simulink model "soc_dvbs2_fpga"  (R2025b)
settings: Solver=FixedStepDiscrete  StartTime=0.0  StopTime=0  RelTol=1e-3
InitFcn:
  | soc_dvbs2_init;
values from neighbouring files (symbols this model uses):
  Rsym = 4e6    (= 4000000)    [soc_dvbs2_init.m]
  soc_dvbs2_txPacketBits = [1 1 0 1 0 1 1 1 0 1 1 1 ... (2972 elements, 2972x1)]    [soc_dvbs2_txPacketBits.mat]
  syncWord = (dec2bin(hex2dec('AC')) - '0').'    [soc_dvbs2_init.m]
  txDataOut = txobj(frameBits(:))    [soc_dvbs2_init.m]
  txFiltCoeff = txobj.pTxFilterCoeff    [soc_dvbs2_init.m]
undefined symbols (not defined in the file or in its folder): Add, coefficientsLog, coefficientsSqrt1, coefficientsSqrt2, dataBits, designMultirateFIR, noisePow, NumBits1, NumBits2, seedsURNG1, seedsURNG2, Shift, Slope1, Slope2, soc_dvbs2_designFIRFilter, txDataOutS1, txDataOutS10, txDataOutS12, txDataOutS13, txDataOutS14, txDataOutS15, txDataOutS16, txDataOutS18, txDataOutS19, txDataOutS2, txDataOutS20, txDataOutS21, txDataOutS22, txDataOutS24, txDataOutS25, txDataOutS26, txDataOutS27, txDataOutS3, txDataOutS4, txDataOutS5, txDataOutS6, txDataOutS7, txDataOutS8, txDataOutS9
libraries: simulink x214, hdlsllib x211, dspsigops x22, dsphdlfiltering2 x8, dsphdlsigops2 x5, commseqgen3 x5, dsphdlmathfun2 x3, hwlogicconnlib x2, whdledac x2, commhdlcrc x2, whdlutilities x1, whdlmod x1
(part 9 of 12)

== system soc_dvbs2_fpga/DVBS2/DVBS2 TxRx/DVB-S2 HDL Receiver/Synchronizer and PL Header Decoder/Time Frequency and Coarse Phase Synchronizer/Coarse Phase Synchronizer/Coarse Phase Corrector/Reciprocal/Function Impl ==
  switch : Inport
  LUTAddr : Inport  Port=2
  Delay{6..8,10,15..16} (6 alike) : Delay
  Delay9 : Delay  DelayLength=1
  LUT1 : LookupNDDirect  NumberOfTableDimensions=1  Table=LUT(:,1)  DiagnosticForOutOfRangeInput=Error
  LUT2 : LookupNDDirect  NumberOfTableDimensions=1  Table=LUT(:,2)  DiagnosticForOutOfRangeInput=Error
  Multiport Switch : MultiPortSwitch  DataPortOrder=Zero-based contiguous  Inputs=2  zeroidx=on  SaturateOnIntegerOverflow=off  InputSameDT=off
  functionValues : Outport
  wires:
  LUTAddr/1 -> Delay7/1, Delay6/1
  Delay15/1 -> Multiport Switch/2
  Delay16/1 -> Multiport Switch/3
  Delay10/1 -> Multiport Switch/1
  Delay9/1 -> functionValues/1
  LUT2/1 -> Delay15/1
  LUT1/1 -> Delay16/1
  switch/1 -> Delay8/1
  Delay8/1 -> Delay10/1
  Delay7/1 -> LUT2/1
  Delay6/1 -> LUT1/1
  Multiport Switch/1 -> Delay9/1

== system soc_dvbs2_fpga/DVBS2/DVBS2 TxRx/DVB-S2 HDL Receiver/Synchronizer and PL Header Decoder/Time Frequency and Coarse Phase Synchronizer/Fine Frequency Synchronizer/Modified L and R Algorithm/L and R Algorithm 18 point/Compute R(m) for 1 to 6 ==
  z : Inport
  zvalid : Inport  Port=2
  Add2 : Sum  Inputs=++++++
  Compute R(m)_1 : Subsystem  mask{m=m(1), N=config.nPilot}
      mask prompts: m "m value :"; N "N value :"
      mask init:
      | validateattributes(N,{'numeric'},{'finite','positive','integer'})
      | validateattributes(m,{'numeric'},{'finite','positive','integer','>=',1,'<=',N-1})
      | MulDivFactor = fi(1/(N-m),0,16);
  Compute R(m)_2 : Subsystem  mask{m=m(2), N=config.nPilot}
      mask prompts: m "m value :"; N "N value :"
      mask init:
      | validateattributes(N,{'numeric'},{'finite','positive','integer'})
      | validateattributes(m,{'numeric'},{'finite','positive','integer','>=',1,'<=',N-1})
      | MulDivFactor = fi(1/(N-m),0,16);
  Compute R(m)_3 : Subsystem  mask{m=m(3), N=config.nPilot}
      mask prompts: m "m value :"; N "N value :"
      mask init:
      | validateattributes(N,{'numeric'},{'finite','positive','integer'})
      | validateattributes(m,{'numeric'},{'finite','positive','integer','>=',1,'<=',N-1})
      | MulDivFactor = fi(1/(N-m),0,16);
  Compute R(m)_4 : Subsystem  mask{m=m(4), N=config.nPilot}
      mask prompts: m "m value :"; N "N value :"
      mask init:
      | validateattributes(N,{'numeric'},{'finite','positive','integer'})
      | validateattributes(m,{'numeric'},{'finite','positive','integer','>=',1,'<=',N-1})
      | MulDivFactor = fi(1/(N-m),0,16);
  Compute R(m)_5 : Subsystem  mask{m=m(5), N=config.nPilot}
      mask prompts: m "m value :"; N "N value :"
      mask init:
      | validateattributes(N,{'numeric'},{'finite','positive','integer'})
      | validateattributes(m,{'numeric'},{'finite','positive','integer','>=',1,'<=',N-1})
      | MulDivFactor = fi(1/(N-m),0,16);
  Compute R(m)_6 : Subsystem  mask{m=m(6), N=config.nPilot}
      mask prompts: m "m value :"; N "N value :"
      mask init:
      | validateattributes(N,{'numeric'},{'finite','positive','integer'})
      | validateattributes(m,{'numeric'},{'finite','positive','integer','>=',1,'<=',N-1})
      | MulDivFactor = fi(1/(N-m),0,16);
  Delay{1..7} (7 alike) : Delay
  sum : Outport
  wires:
  z/1 -> Compute R(m)_1/1(z), Compute R(m)_5/1(z), Compute R(m)_6/1(z), Compute R(m)_4/1(z), Compute R(m)_3/1(z), Compute R(m)_2/1(z)
  Delay3/1 -> Add2/1
  Delay7/1 -> sum/1
  Delay6/1 -> Add2/6
  Delay5/1 -> Add2/5
  Delay4/1 -> Add2/4
  Delay2/1 -> Add2/3
  Delay1/1 -> Add2/2
  zvalid/1 -> Compute R(m)_1/2(zvalid), Compute R(m)_5/2(zvalid), Compute R(m)_6/2(zvalid), Compute R(m)_4/2(zvalid), Compute R(m)_3/2(zvalid), Compute R(m)_2/2(zvalid)
  Compute R(m)_6/1(Out1) -> Delay6/1
  Compute R(m)_5/1(Out1) -> Delay5/1
  Compute R(m)_4/1(Out1) -> Delay4/1
  Compute R(m)_3/1(Out1) -> Delay2/1
  Compute R(m)_2/1(Out1) -> Delay1/1
  Compute R(m)_1/1(Out1) -> Delay3/1
  Add2/1 -> Delay7/1

== system soc_dvbs2_fpga/DVBS2/DVBS2 TxRx/DVB-S2 HDL Receiver/Synchronizer and PL Header Decoder/Time Frequency and Coarse Phase Synchronizer/Fine Frequency Synchronizer/Modified L and R Algorithm/L and R Algorithm 18 point/Compute R(m) for 13 to 18 ==
  z : Inport
  zvalid : Inport  Port=2
  Add2 : Sum  Inputs=++++++
  Compute R(m)_1 : Subsystem  mask{m=m(1), N=config.nPilot}
      mask prompts: m "m value :"; N "N value :"
      mask init:
      | validateattributes(N,{'numeric'},{'finite','positive','integer'})
      | validateattributes(m,{'numeric'},{'finite','positive','integer','>=',1,'<=',N-1})
      | MulDivFactor = fi(1/(N-m),0,16);
  Compute R(m)_2 : Subsystem  mask{m=m(2), N=config.nPilot}
      mask prompts: m "m value :"; N "N value :"
      mask init:
      | validateattributes(N,{'numeric'},{'finite','positive','integer'})
      | validateattributes(m,{'numeric'},{'finite','positive','integer','>=',1,'<=',N-1})
      | MulDivFactor = fi(1/(N-m),0,16);
  Compute R(m)_3 : Subsystem  mask{m=m(3), N=config.nPilot}
      mask prompts: m "m value :"; N "N value :"
      mask init:
      | validateattributes(N,{'numeric'},{'finite','positive','integer'})
      | validateattributes(m,{'numeric'},{'finite','positive','integer','>=',1,'<=',N-1})
      | MulDivFactor = fi(1/(N-m),0,16);
  Compute R(m)_4 : Subsystem  mask{m=m(4), N=config.nPilot}
      mask prompts: m "m value :"; N "N value :"
      mask init:
      | validateattributes(N,{'numeric'},{'finite','positive','integer'})
      | validateattributes(m,{'numeric'},{'finite','positive','integer','>=',1,'<=',N-1})
      | MulDivFactor = fi(1/(N-m),0,16);
  Compute R(m)_5 : Subsystem  mask{m=m(5), N=config.nPilot}
      mask prompts: m "m value :"; N "N value :"
      mask init:
      | validateattributes(N,{'numeric'},{'finite','positive','integer'})
      | validateattributes(m,{'numeric'},{'finite','positive','integer','>=',1,'<=',N-1})
      | MulDivFactor = fi(1/(N-m),0,16);
  Compute R(m)_6 : Subsystem  mask{m=m(6), N=config.nPilot}
      mask prompts: m "m value :"; N "N value :"
      mask init:
      | validateattributes(N,{'numeric'},{'finite','positive','integer'})
      | validateattributes(m,{'numeric'},{'finite','positive','integer','>=',1,'<=',N-1})
      | MulDivFactor = fi(1/(N-m),0,16);
  Delay{1..7} (7 alike) : Delay
  sum : Outport
  wires:
  z/1 -> Compute R(m)_1/1(z), Compute R(m)_5/1(z), Compute R(m)_6/1(z), Compute R(m)_4/1(z), Compute R(m)_3/1(z), Compute R(m)_2/1(z)
  Delay3/1 -> Add2/1
  Delay7/1 -> sum/1
  Delay6/1 -> Add2/6
  Delay5/1 -> Add2/5
  Delay4/1 -> Add2/4
  Delay2/1 -> Add2/3
  Delay1/1 -> Add2/2
  zvalid/1 -> Compute R(m)_1/2(zvalid), Compute R(m)_5/2(zvalid), Compute R(m)_6/2(zvalid), Compute R(m)_4/2(zvalid), Compute R(m)_3/2(zvalid), Compute R(m)_2/2(zvalid)
  Compute R(m)_6/1(Out1) -> Delay6/1
  Compute R(m)_5/1(Out1) -> Delay5/1
  Compute R(m)_4/1(Out1) -> Delay4/1
  Compute R(m)_3/1(Out1) -> Delay2/1
  Compute R(m)_2/1(Out1) -> Delay1/1
  Compute R(m)_1/1(Out1) -> Delay3/1
  Add2/1 -> Delay7/1

== system soc_dvbs2_fpga/DVBS2/DVBS2 TxRx/DVB-S2 HDL Receiver/Synchronizer and PL Header Decoder/Time Frequency and Coarse Phase Synchronizer/Fine Frequency Synchronizer/Modified L and R Algorithm/L and R Algorithm 18 point/Compute R(m) for 7 to 12 ==
  z : Inport
  zvalid : Inport  Port=2
  Add2 : Sum  Inputs=++++++
  Compute R(m)_1 : Subsystem  mask{m=m(1), N=config.nPilot}
      mask prompts: m "m value :"; N "N value :"
      mask init:
      | validateattributes(N,{'numeric'},{'finite','positive','integer'})
      | validateattributes(m,{'numeric'},{'finite','positive','integer','>=',1,'<=',N-1})
      | MulDivFactor = fi(1/(N-m),0,16);
  Compute R(m)_2 : Subsystem  mask{m=m(2), N=config.nPilot}
      mask prompts: m "m value :"; N "N value :"
      mask init:
      | validateattributes(N,{'numeric'},{'finite','positive','integer'})
      | validateattributes(m,{'numeric'},{'finite','positive','integer','>=',1,'<=',N-1})
      | MulDivFactor = fi(1/(N-m),0,16);
  Compute R(m)_3 : Subsystem  mask{m=m(3), N=config.nPilot}
      mask prompts: m "m value :"; N "N value :"
      mask init:
      | validateattributes(N,{'numeric'},{'finite','positive','integer'})
      | validateattributes(m,{'numeric'},{'finite','positive','integer','>=',1,'<=',N-1})
      | MulDivFactor = fi(1/(N-m),0,16);
  Compute R(m)_4 : Subsystem  mask{m=m(4), N=config.nPilot}
      mask prompts: m "m value :"; N "N value :"
      mask init:
      | validateattributes(N,{'numeric'},{'finite','positive','integer'})
      | validateattributes(m,{'numeric'},{'finite','positive','integer','>=',1,'<=',N-1})
      | MulDivFactor = fi(1/(N-m),0,16);
  Compute R(m)_5 : Subsystem  mask{m=m(5), N=config.nPilot}
      mask prompts: m "m value :"; N "N value :"
      mask init:
      | validateattributes(N,{'numeric'},{'finite','positive','integer'})
      | validateattributes(m,{'numeric'},{'finite','positive','integer','>=',1,'<=',N-1})
      | MulDivFactor = fi(1/(N-m),0,16);
  Compute R(m)_6 : Subsystem  mask{m=m(6), N=config.nPilot}
      mask prompts: m "m value :"; N "N value :"
      mask init:
      | validateattributes(N,{'numeric'},{'finite','positive','integer'})
      | validateattributes(m,{'numeric'},{'finite','positive','integer','>=',1,'<=',N-1})
      | MulDivFactor = fi(1/(N-m),0,16);
  Delay{1..7} (7 alike) : Delay
  sum : Outport
  wires:
  Add2/1 -> Delay7/1
  Compute R(m)_1/1(Out1) -> Delay3/1
  Compute R(m)_2/1(Out1) -> Delay1/1
  Compute R(m)_3/1(Out1) -> Delay2/1
  Compute R(m)_4/1(Out1) -> Delay4/1
  Compute R(m)_5/1(Out1) -> Delay5/1
  Compute R(m)_6/1(Out1) -> Delay6/1
  zvalid/1 -> Compute R(m)_2/2(zvalid), Compute R(m)_3/2(zvalid), Compute R(m)_4/2(zvalid), Compute R(m)_6/2(zvalid), Compute R(m)_5/2(zvalid), Compute R(m)_1/2(zvalid)
  Delay1/1 -> Add2/2
  Delay2/1 -> Add2/3
  Delay4/1 -> Add2/4
  Delay5/1 -> Add2/5
  Delay6/1 -> Add2/6
  Delay7/1 -> sum/1
  Delay3/1 -> Add2/1
  z/1 -> Compute R(m)_2/1(z), Compute R(m)_3/1(z), Compute R(m)_4/1(z), Compute R(m)_6/1(z), Compute R(m)_5/1(z), Compute R(m)_1/1(z)

== system soc_dvbs2_fpga/DVBS2/DVBS2 TxRx/DVB-S2 HDL Receiver/Synchronizer and PL Header Decoder/Time Frequency and Coarse Phase Synchronizer/Time and Coarse Frequency Synchronizer/Coarse Frequency Estimator/Frequency Error Detector/Complex Multiplier ==
  In1 : Inport
  In2 : Inport  Port=2
  AddADn : Sum  Inputs=++|  OutDataTypeStr=Inherit: Same as first input
  AddAUp : Sum  Inputs=|+-  OutDataTypeStr=Inherit: Same as first input
  AddBCtr : Sum  Inputs=+|+
  AddBDn : Sum  Inputs=|+-
  AddBUp : Sum  Inputs=++|
  Complex to Real-Imag : ComplexToRealImag
  Complex to Real-Imag1 : ComplexToRealImag
  Delay{1..5,8..20} (18 alike) : Delay  DelayLength=1
  Delay{6..7,21..27} (9 alike) : Delay
  Product : Product
  Product1 : Product
  Product2 : Product
  Real-Imag to Complex : RealImagToComplex
  Out1 : Outport  VectorParamsAs1DForOutWhenUnconnected=off
  wires:
  Delay27/1 -> Delay18/1
  Delay26/1 -> Delay17/1
  Delay25/1 -> Delay16/1
  Delay24/1 -> Product2/2
  Delay23/1 -> Product2/1
  Delay22/1 -> Product1/2
  Delay21/1 -> Product1/1
  Delay7/1 -> Product/2
  Delay6/1 -> Product/1
  Delay13/1 -> AddBCtr/2, Delay4/1
  Delay12/1 -> Delay3/1
  Delay11/1 -> AddBCtr/1, Delay1/1
  In2/1 -> Complex to Real-Imag1/1
  In1/1 -> Complex to Real-Imag/1
  Product2/1 -> Delay27/1
  Product1/1 -> Delay26/1
  Product/1 -> Delay25/1
  Complex to Real-Imag1/1 -> [RE2]
  Complex to Real-Imag1/2 -> [IM2]
  [IM2] -> Delay10/1
  [RE2] -> Delay9/1
  Complex to Real-Imag/1 -> Delay11/1
  AddBUp/1 -> Delay8/1
  [RE2] -> Delay14/1
  [IM2] -> Delay15/1
  AddBDn/1 -> Delay5/1
  Complex to Real-Imag/2 -> Delay13/1
  AddBCtr/1 -> Delay2/1
  [IM2] -> Delay12/1
  AddADn/1 -> Delay20/1
  AddAUp/1 -> Delay19/1
  Real-Imag to Complex/1 -> Out1/1
  Delay5/1 -> Delay24/1
  Delay4/1 -> Delay23/1
  Delay3/1 -> Delay22/1
  Delay2/1 -> Delay21/1
  Delay8/1 -> Delay6/1
  Delay9/1 -> AddBUp/1
  Delay10/1 -> AddBUp/2
  Delay14/1 -> AddBDn/1
  Delay15/1 -> AddBDn/2
  Delay16/1 -> AddAUp/1
  Delay17/1 -> AddADn/1, AddAUp/2
  Delay18/1 -> AddADn/2
  Delay19/1 -> Real-Imag to Complex/1
  Delay20/1 -> Real-Imag to Complex/2
  Delay1/1 -> Delay7/1

== system soc_dvbs2_fpga/DVBS2/DVBS2 TxRx/DVB-S2 HDL Receiver/Synchronizer and PL Header Decoder/Time Frequency and Coarse Phase Synchronizer/Time and Coarse Frequency Synchronizer/Frame Synchronizer/Correlator/Moving Sum ==
  scaled1 : Inport
  scaled2 : Inport  Port=2
  validIn : Inport  Port=3
  Add : Sum  Inputs=|+-  OutDataTypeStr=Inherit: Same as first input
  Add1 : Sum  Inputs=|++  OutDataTypeStr=Inherit: Same as first input
  Add2 : Sum  Inputs=|+-  OutDataTypeStr=Inherit: Same as first input
  Add3 : Sum  Inputs=|++  OutDataTypeStr=Inherit: Same as first input
  Delay : Delay  DelayLength=length(config.refSOF)  ShowEnablePort=on
      settings: InputPortMap=u0,e6
  Delay1 : Delay  DelayLength=length(config.refPLSC)  ShowEnablePort=on
      settings: InputPortMap=u0,e6
  Delay11 : Delay  DelayLength=70
  Delay14 : Delay  DelayLength=1  ShowEnablePort=on
      settings: InputPortMap=u0,e6
  Delay2 : Delay  DelayLength=1  ShowEnablePort=on
      settings: InputPortMap=u0,e6
  Delay3 : Delay  DelayLength=length(config.refPLSC) - length(config.refSOF)  ShowEnablePort=on
      settings: InputPortMap=u0,e6
  Delay4 : Delay  DelayLength=70
  E1 : Outport
  E2 : Outport  Port=2
  wires:
  Delay4/1 -> E2/1
  Delay11/1 -> E1/1
  Delay3/1 -> Delay11/1
  Delay2/1 -> Add3/2
  scaled1/1 -> Add/1, Delay/1
  Delay1/1 -> Add2/2
  Add2/1 -> Add3/1
  Delay14/1 -> Add1/2
  Delay/1 -> Add/2
  Add3/1 -> Delay4/1, Delay2/1
  validIn/1 -> Delay14/2, Delay3/2, Delay/2, Delay1/2, Delay2/2
  Add1/1 -> Delay14/1, Delay3/1
  scaled2/1 -> Delay1/1, Add2/1
  Add/1 -> Add1/1

== system soc_dvbs2_fpga/DVBS2/DVBS2 TxRx/DVB-S2 HDL Receiver/Synchronizer and PL Header Decoder/Time Frequency and Coarse Phase Synchronizer/Time and Coarse Frequency Synchronizer/Frame Synchronizer/Correlator/PLSC Correlator ==
  dataIn : Inport
  validIn : Inport  Port=2
  Data Type Conversion : DataTypeConversion  OutDataTypeStr=fixdt(1,18,15)  SaturateOnIntegerOverflow=off  RndMeth=Floor
  Delay : Delay  DelayLength=partlySerialExtraDelay
  Delay1 : Delay  DelayLength=partlySerialExtraDelay
  Delay3 : Delay  DelayLength=adjustDelay
  Discrete FIR Filter : dsphdlfiltering2/Discrete FIR Filter  NumeratorSource=Property  Numerator=coefs  NumeratorPrototype=[]  FilterStructure=Partly serial systolic  SerializationOption=Minimum number of cycles between valid input samples  NumCycles=shareFactor  NumberOfMultipliers=2  SimulateUsing=Code generation  roundingMode=Floor  overflowMode=off  CoefficientsDataTypeStr=Inherit: Same word length as input  OutputDataTypeStr=Inherit: Same word length as input  ResetInputPort=off  HDLGlobalReset=off  CoeffMultiplier=Multiplier  UseMultForPow2Coeff=on  FrameInputSymmOptim=off
  Downsample : DownSample  N=shareFactor  RateOptions=Allow multirate processing
  Terminator : Terminator
  Unit Delay Enabled Synchronous : hdlsllib/Discrete/Unit Delay Enabled Synchronous  InitialCondition=0.0  SampleTime=-1
  Upsample : dspsigops/Upsample  FactorSource=Dialog parameter  N=shareFactor  Nmax=16  phase=0  RateOptions=Allow multirate processing  ic=0  mode=Unused parameter value
  Upsample1 : dspsigops/Upsample  FactorSource=Dialog parameter  N=shareFactor  Nmax=16  phase=0  RateOptions=Allow multirate processing  ic=0  mode=Unused parameter value
  dataOut : Outport
  wires:
  Downsample/1 -> Delay3/1
  Delay1/1 -> Unit Delay Enabled Synchronous/2
  Upsample1/1 -> Discrete FIR Filter/2
  Discrete FIR Filter/1 -> Delay/1
  Delay/1 -> Unit Delay Enabled Synchronous/1
  Discrete FIR Filter/2 -> Delay1/1
  Unit Delay Enabled Synchronous/1 -> Downsample/1
  Upsample/1 -> Discrete FIR Filter/1
  dataIn/1 -> Upsample/1
  validIn/1 -> Upsample1/1
  Delay3/1 -> Data Type Conversion/1
  Discrete FIR Filter/3 -> Terminator/1
  Data Type Conversion/1 -> dataOut/1

== system soc_dvbs2_fpga/DVBS2/DVBS2 TxRx/DVB-S2 HDL Receiver/Synchronizer and PL Header Decoder/Time Frequency and Coarse Phase Synchronizer/Time and Coarse Frequency Synchronizer/Frame Synchronizer/Correlator/SOF Correlator ==
  dataIn : Inport
  validIn : Inport  Port=2
  Data Type Conversion : DataTypeConversion  OutDataTypeStr=fixdt(1,18,15)  SaturateOnIntegerOverflow=off  RndMeth=Floor
  Delay : Delay  DelayLength=partlySerialExtraDelay
  Delay1 : Delay  DelayLength=partlySerialExtraDelay
  Delay3 : Delay  DelayLength=adjustDelay
  Discrete FIR Filter : dsphdlfiltering2/Discrete FIR Filter  NumeratorSource=Property  Numerator=coefs  NumeratorPrototype=[]  FilterStructure=Partly serial systolic  SerializationOption=Minimum number of cycles between valid input samples  NumCycles=shareFactor  NumberOfMultipliers=2  SimulateUsing=Code generation  roundingMode=Floor  overflowMode=off  CoefficientsDataTypeStr=Inherit: Same word length as input  OutputDataTypeStr=Inherit: Same word length as input  ResetInputPort=off  HDLGlobalReset=off  CoeffMultiplier=Multiplier  UseMultForPow2Coeff=on  FrameInputSymmOptim=off
  Downsample : DownSample  N=shareFactor  RateOptions=Allow multirate processing
  Terminator : Terminator
  Unit Delay Enabled Synchronous : hdlsllib/Discrete/Unit Delay Enabled Synchronous  InitialCondition=0.0  SampleTime=-1
  Upsample : dspsigops/Upsample  FactorSource=Dialog parameter  N=shareFactor  Nmax=16  phase=0  RateOptions=Allow multirate processing  ic=0  mode=Unused parameter value
  Upsample1 : dspsigops/Upsample  FactorSource=Dialog parameter  N=shareFactor  Nmax=16  phase=0  RateOptions=Allow multirate processing  ic=0  mode=Unused parameter value
  dataOut : Outport
  wires:
  Data Type Conversion/1 -> dataOut/1
  Discrete FIR Filter/3 -> Terminator/1
  Delay3/1 -> Data Type Conversion/1
  validIn/1 -> Upsample1/1
  dataIn/1 -> Upsample/1
  Upsample/1 -> Discrete FIR Filter/1
  Unit Delay Enabled Synchronous/1 -> Downsample/1
  Discrete FIR Filter/2 -> Delay1/1
  Delay/1 -> Unit Delay Enabled Synchronous/1
  Discrete FIR Filter/1 -> Delay/1
  Upsample1/1 -> Discrete FIR Filter/2
  Delay1/1 -> Unit Delay Enabled Synchronous/2
  Downsample/1 -> Delay3/1

== system soc_dvbs2_fpga/DVBS2/DVBS2 TxRx/DVB-S2 HDL Receiver/Synchronizer and PL Header Decoder/Time Frequency and Coarse Phase Synchronizer/Time and Coarse Frequency Synchronizer/Frame Synchronizer/Pilot and Sync Pulse Indicator/No HDL Correlation Value ==
  PeakValueWithPilots : Inport
  In1 : Inport  Port=2
  PeakValueWithoutPilots : Inport  Port=3
  Delay27 : Delay  DelayLength=1
  Delay28 : Delay  DelayLength=1
  Switch : Switch  Criteria=u2 ~= 0  SaturateOnIntegerOverflow=off  InputSameDT=off
  Terminator : Terminator
  wires:
  PeakValueWithoutPilots/1 -> Delay28/1
  Delay28/1 -> Switch/3
  In1/1 -> Switch/2
  Delay27/1 -> Switch/1
  Switch/1 -> Terminator/1
  PeakValueWithPilots/1 -> Delay27/1

== system soc_dvbs2_fpga/DVBS2/DVBS2 TxRx/DVB-S2 HDL Receiver/Synchronizer and PL Header Decoder/Time Frequency and Coarse Phase Synchronizer/Time and Coarse Frequency Synchronizer/PL Data Descrambler and Pilot Valid Indicator/PL Data Descrambler/PL Scrambler Gold Sequence Generator ==
  reset : Inport
  validIn : Inport  Port=2
  Bit Concat : hdlsllib/Logic and Bit Operations/Bit Concat  numInputs=2
  Delay{,3..4,10,12..15} (8 alike) : Delay  DelayLength=1
  Delay{1..2,5..9,11} (8 alike) : Delay
  Logical Operator : Logic  Operator=XOR  AllPortsSameDT=off  OutDataTypeStr=boolean
  Logical Operator1 : Logic  Operator=XOR  AllPortsSameDT=off  OutDataTypeStr=boolean
  Logical Operator2 : Logic  Operator=OR  AllPortsSameDT=off  OutDataTypeStr=boolean
  Subsystem : Subsystem
  dataOut : Outport
  validOut : Outport  Port=2
  wires:
  Delay15/1 -> validOut/1
  Delay14/1 -> dataOut/1
  Delay13/1 -> Delay15/1
  Delay12/1 -> Bit Concat/2
  Delay10/1 -> Bit Concat/1
  Delay9/1 -> Logical Operator/2
  Delay8/1 -> Logical Operator/1
  Delay7/1 -> Logical Operator1/2
  Delay6/1 -> Logical Operator1/1
  Delay5/1 -> Delay13/1
  Delay4/1 -> Delay2/1, Logical Operator2/1
  Delay3/1 -> Delay/1
  Delay2/1 -> Delay5/1
  Delay1/1 -> Subsystem/Enable
  Delay11/1 -> Subsystem/1(reset)
  Delay/1 -> Logical Operator2/2, Delay11/1
  validIn/1 -> Delay4/1
  Logical Operator1/1 -> Delay10/1
  Logical Operator/1 -> Delay12/1
  Bit Concat/1 -> Delay14/1
  reset/1 -> Delay3/1
  Subsystem/1(xMnp131072) -> Delay6/1
  Subsystem/2(yM131072) -> Delay7/1
  Subsystem/3(xMn) -> Delay8/1
  Subsystem/4(yM0) -> Delay9/1
  Logical Operator2/1 -> Delay1/1

== system soc_dvbs2_fpga/DVBS2/DVBS2 TxRx/DVB-S2 HDL Receiver/Synchronizer and PL Header Decoder/Time Frequency and Coarse Phase Synchronizer/Time and Coarse Frequency Synchronizer/Symbol Synchronizer/Gardner TED/GTED ==
  In1 : Inport
  Add : Sum
  Add1 : Sum  Inputs=+-
  Add2 : Sum  Inputs=+-
  Complex to Real-Imag : ComplexToRealImag
  Delay{,1..7} (8 alike) : Delay  DelayLength=1
  Delay{8..13} (6 alike) : Delay
  Product : Product
  Product1 : Product
  Out1 : Outport
  wires:
  Delay13/1 -> Add/2
  Delay12/1 -> Product1/2
  Delay11/1 -> Product1/1
  Delay10/1 -> Add/1
  Delay9/1 -> Product/2
  Delay8/1 -> Product/1
  Complex to Real-Imag/2 -> Delay4/1, Add2/2
  Delay7/1 -> Add2/1
  Delay4/1 -> Delay5/1
  Delay6/1 -> Delay7/1
  Add2/1 -> Delay12/1
  Delay5/1 -> Delay6/1, Delay11/1
  Delay1/1 -> Delay8/1, Delay2/1
  Add1/1 -> Delay9/1
  Delay2/1 -> Delay3/1
  Delay/1 -> Delay1/1
  Delay3/1 -> Add1/1
  Complex to Real-Imag/1 -> Delay/1, Add1/2
  In1/1 -> Complex to Real-Imag/1
  Add/1 -> Out1/1
  Product1/1 -> Delay13/1
  Product/1 -> Delay10/1

== system soc_dvbs2_fpga/DVBS2/DVBS2 TxRx/DVB-S2 HDL Receiver/Synchronizer and PL Header Decoder/Time Frequency and Coarse Phase Synchronizer/Time and Coarse Frequency Synchronizer/Symbol Synchronizer/Rate Handle/FIFO ==
  data : Inport
  push : Inport  Port=2
  pop : Inport  Port=3
  Delay1 : Delay  DelayLength=1
  Delay2 : Delay  DelayLength=1
  HDL Counter : hdlsllib/Sources/HDL Counter  CountType=Count limited  CountInit=0  CountStep=1  CountMax=1024-1  CountFromType=Initial value  CountFrom=0  CountResetPort=off  CountLoadPort=off  CountEnbPort=on  CountDirPort=off  CountHitOutputPort=off  CountDataType=Unsigned  CountWordLen=nextpow2(1024-1)  CountFracLen=0  CountSampTime=1
  HDL Counter1 : hdlsllib/Sources/HDL Counter  CountType=Count limited  CountInit=0  CountStep=1  CountMax=1024 - 1  CountFromType=Initial value  CountFrom=0  CountResetPort=off  CountLoadPort=off  CountEnbPort=on  CountDirPort=off  CountHitOutputPort=off  CountDataType=Unsigned  CountWordLen=nextpow2(1024-1)  CountFracLen=0  CountSampTime=1
  Logical Operator : Logic  AllPortsSameDT=off  OutDataTypeStr=boolean
  Logical Operator1 : Logic  Operator=OR  AllPortsSameDT=off  OutDataTypeStr=boolean
  Logical Operator2 : Logic  Operator=NOT  AllPortsSameDT=off  OutDataTypeStr=boolean
  Logical Operator3 : Logic  AllPortsSameDT=off  OutDataTypeStr=boolean
  MATLAB Function : MATLAB Function  TreatAsAtomicUnit=on
  Simple Dual Port RAM : hdlsllib/HDL RAMs/Simple Dual Port RAM  ram_size=nextpow2(1024-1)
  out : Outport
  outValid : Outport  Port=2
  wires:
  pop/1 -> Logical Operator3/2
  Logical Operator2/1 -> Logical Operator3/1
  Delay2/1 -> Logical Operator2/1
  Logical Operator/1 -> Logical Operator1/1
  Logical Operator1/1 -> HDL Counter1/1
  Delay1/1 -> Logical Operator/2
  MATLAB Function/2(empty) -> Delay2/1
  MATLAB Function/1(full) -> Delay1/1
  Simple Dual Port RAM/1 -> out/1
  HDL Counter1/1 -> Simple Dual Port RAM/4
  Logical Operator3/1 -> Logical Operator1/2, MATLAB Function/2(rd), outValid/1
  HDL Counter/1 -> Simple Dual Port RAM/2
  push/1 -> Logical Operator/1, Simple Dual Port RAM/3, HDL Counter/1, MATLAB Function/1(wr)
  data/1 -> Simple Dual Port RAM/1

== system soc_dvbs2_fpga/DVBS2/DVBS2 TxRx/DVB-S2 HDL Receiver/Synchronizer and PL Header Decoder/Time Frequency and Coarse Phase Synchronizer/Fine Frequency Synchronizer/Modified L and R Algorithm/L and R Algorithm 18 point/Compute R(m) for 1 to 6/Compute R(m)_1 ==
  z : Inport
  zvalid : Inport  Port=2
  Add3 : Sum  Inputs=++|  OutDataTypeStr=Inherit: Inherit via back propagation
  Compare To Constant : simulink/Logic and Bit Operations/Compare To Constant  relop=>=  const=m  OutDataTypeStr=boolean
  Compare To Constant2 : simulink/Logic and Bit Operations/Compare To Constant  relop===  const=N - 1  OutDataTypeStr=boolean
  Complex Multiplier : Subsystem  VariantControl=Use 3 multipliers and 5 adders
      mask Display: disp(['Complex Multiplier' newline 'Latency = 8']);
  Data Type Duplicate : DataTypeDuplicate
  Data Type Conversion : DataTypeConversion  Commented=through  OutDataTypeStr=fixdt(1,28,17)  SaturateOnIntegerOverflow=off  RndMeth=Floor
  Delay : Delay  DelayLength=m
  Delay{1..2,7..9,11..12,14..15} (9 alike) : Delay  DelayLength=1
  Delay{3..6,10,13,16..26} (17 alike) : Delay
  Delay{27..30} (4 alike) : Delay  DelayLength=8
  Gain : Gain  Gain=MulDivFactor  ParamDataTypeStr=Inherit: Inherit from 'Gain'  OutDataTypeStr=Inherit: Same as input
  HDL Counter : hdlsllib/Sources/HDL Counter  CountType=Count limited  CountInit=0  CountStep=1  CountMax=N-1  CountFromType=Initial value  CountFrom=0  CountResetPort=off  CountLoadPort=off  CountEnbPort=on  CountDirPort=off  CountHitOutputPort=off  CountDataType=Unsigned  CountWordLen=nextpow2(N-1)  CountFracLen=0  CountSampTime=1
  Logical Operator : Logic  AllPortsSameDT=off  OutDataTypeStr=boolean
  Logical Operator1 : Logic  AllPortsSameDT=off  OutDataTypeStr=boolean
  Math Function : Math  Operator=conj
  Unit Delay Enabled Synchronous : hdlsllib/Discrete/Unit Delay Enabled Synchronous  InitialCondition=0.0  SampleTime=-1
  Unit Delay Enabled Resettable Synchronous : hdlsllib/Discrete/Unit Delay Enabled Resettable Synchronous  InitialCondition=0.0  SampleTime=-1
  Out1 : Outport
  wires:
  Data Type Conversion/1 -> Delay13/1
  Delay30/1 -> Delay20/1
  Delay29/1 -> Compare To Constant2/1
  Delay28/1 -> Compare To Constant/1
  Delay27/1 -> Delay17/1
  Delay13/1 -> Delay21/1
  Complex Multiplier/1(Out1) -> Data Type Conversion/1
  Delay26/1 -> Delay1/1
  Logical Operator/1 -> Delay25/1
  Delay24/1 -> Unit Delay Enabled Resettable Synchronous/2
  Delay23/1 -> Delay24/1
  Delay22/1 -> Add3/2, Data Type Duplicate/1
  Delay21/1 -> Gain/1
  Gain/1 -> Delay22/1
  Unit Delay Enabled Synchronous/1 -> Out1/1
  Delay20/1 -> Logical Operator/2
  Delay19/1 -> Logical Operator/1
  Delay18/1 -> Logical Operator1/2
  Delay17/1 -> Logical Operator1/1
  Delay16/1 -> Delay30/1
  Delay15/1 -> Delay16/1
  Delay12/1 -> Delay6/1
  Delay11/1 -> Delay5/1
  Delay10/1 -> Delay27/1
  Delay9/1 -> Delay10/1
  Delay8/1 -> Delay4/1
  Delay7/1 -> Delay3/1
  Delay6/1 -> Delay29/1
  Delay5/1 -> Delay28/1
  Delay4/1 -> Complex Multiplier/2(In2)
  Delay3/1 -> Complex Multiplier/1(In1)
  Delay2/1 -> Delay/1, Delay7/1
  Delay14/1 -> HDL Counter/1, Delay15/1, Delay9/1
  Math Function/1 -> Delay8/1
  z/1 -> Delay2/1
  Delay/1 -> Math Function/1
  Delay1/1 -> Unit Delay Enabled Resettable Synchronous/3, Unit Delay Enabled Synchronous/2
  Unit Delay Enabled Resettable Synchronous/1 -> Add3/1, Unit Delay Enabled Synchronous/1
  zvalid/1 -> Delay14/1
  Delay25/1 -> Delay26/1
  Compare To Constant2/1 -> Delay19/1
  Compare To Constant/1 -> Delay18/1
  HDL Counter/1 -> Delay12/1, Delay11/1
  Add3/1 -> Unit Delay Enabled Resettable Synchronous/1, Data Type Duplicate/2
  Logical Operator1/1 -> Delay23/1

== system soc_dvbs2_fpga/DVBS2/DVBS2 TxRx/DVB-S2 HDL Receiver/Synchronizer and PL Header Decoder/Time Frequency and Coarse Phase Synchronizer/Fine Frequency Synchronizer/Modified L and R Algorithm/L and R Algorithm 18 point/Compute R(m) for 1 to 6/Compute R(m)_2 ==
  z : Inport
  zvalid : Inport  Port=2
  Add3 : Sum  Inputs=++|  OutDataTypeStr=Inherit: Inherit via back propagation
  Compare To Constant : simulink/Logic and Bit Operations/Compare To Constant  relop=>=  const=m  OutDataTypeStr=boolean
  Compare To Constant2 : simulink/Logic and Bit Operations/Compare To Constant  relop===  const=N - 1  OutDataTypeStr=boolean
  Complex Multiplier : Subsystem  VariantControl=Use 3 multipliers and 5 adders
      mask Display: disp(['Complex Multiplier' newline 'Latency = 8']);
  Data Type Duplicate : DataTypeDuplicate
  Data Type Conversion : DataTypeConversion  Commented=through  OutDataTypeStr=fixdt(1,28,17)  SaturateOnIntegerOverflow=off  RndMeth=Floor
  Delay : Delay  DelayLength=m
  Delay{1..2,7..9,11..12,14..15} (9 alike) : Delay  DelayLength=1
  Delay{3..6,10,13,16..26} (17 alike) : Delay
  Delay{27..30} (4 alike) : Delay  DelayLength=8
  Gain : Gain  Gain=MulDivFactor  ParamDataTypeStr=Inherit: Inherit from 'Gain'  OutDataTypeStr=Inherit: Same as input
  HDL Counter : hdlsllib/Sources/HDL Counter  CountType=Count limited  CountInit=0  CountStep=1  CountMax=N-1  CountFromType=Initial value  CountFrom=0  CountResetPort=off  CountLoadPort=off  CountEnbPort=on  CountDirPort=off  CountHitOutputPort=off  CountDataType=Unsigned  CountWordLen=nextpow2(N-1)  CountFracLen=0  CountSampTime=1
  Logical Operator : Logic  AllPortsSameDT=off  OutDataTypeStr=boolean
  Logical Operator1 : Logic  AllPortsSameDT=off  OutDataTypeStr=boolean
  Math Function : Math  Operator=conj
  Unit Delay Enabled Synchronous : hdlsllib/Discrete/Unit Delay Enabled Synchronous  InitialCondition=0.0  SampleTime=-1
  Unit Delay Enabled Resettable Synchronous : hdlsllib/Discrete/Unit Delay Enabled Resettable Synchronous  InitialCondition=0.0  SampleTime=-1
  Out1 : Outport
  wires:
  Data Type Conversion/1 -> Delay13/1
  Logical Operator1/1 -> Delay23/1
  Add3/1 -> Data Type Duplicate/2, Unit Delay Enabled Resettable Synchronous/1
  HDL Counter/1 -> Delay11/1, Delay12/1
  Compare To Constant/1 -> Delay18/1
  Compare To Constant2/1 -> Delay19/1
  Delay25/1 -> Delay26/1
  zvalid/1 -> Delay14/1
  Unit Delay Enabled Resettable Synchronous/1 -> Unit Delay Enabled Synchronous/1, Add3/1
  Delay1/1 -> Unit Delay Enabled Synchronous/2, Unit Delay Enabled Resettable Synchronous/3
  Delay/1 -> Math Function/1
  z/1 -> Delay2/1
  Math Function/1 -> Delay8/1
  Delay14/1 -> Delay9/1, Delay15/1, HDL Counter/1
  Delay2/1 -> Delay7/1, Delay/1
  Delay3/1 -> Complex Multiplier/1(In1)
  Delay4/1 -> Complex Multiplier/2(In2)
  Delay5/1 -> Delay28/1
  Delay6/1 -> Delay29/1
  Delay7/1 -> Delay3/1
  Delay8/1 -> Delay4/1
  Delay9/1 -> Delay10/1
  Delay10/1 -> Delay27/1
  Delay11/1 -> Delay5/1
  Delay12/1 -> Delay6/1
  Delay15/1 -> Delay16/1
  Delay16/1 -> Delay30/1
  Delay17/1 -> Logical Operator1/1
  Delay18/1 -> Logical Operator1/2
  Delay19/1 -> Logical Operator/1
  Delay20/1 -> Logical Operator/2
  Unit Delay Enabled Synchronous/1 -> Out1/1
  Gain/1 -> Delay22/1
  Delay21/1 -> Gain/1
  Delay22/1 -> Data Type Duplicate/1, Add3/2
  Delay23/1 -> Delay24/1
  Delay24/1 -> Unit Delay Enabled Resettable Synchronous/2
  Logical Operator/1 -> Delay25/1
  Delay26/1 -> Delay1/1
  Complex Multiplier/1(Out1) -> Data Type Conversion/1
  Delay13/1 -> Delay21/1
  Delay27/1 -> Delay17/1
  Delay28/1 -> Compare To Constant/1
  Delay29/1 -> Compare To Constant2/1
  Delay30/1 -> Delay20/1

== system soc_dvbs2_fpga/DVBS2/DVBS2 TxRx/DVB-S2 HDL Receiver/Synchronizer and PL Header Decoder/Time Frequency and Coarse Phase Synchronizer/Fine Frequency Synchronizer/Modified L and R Algorithm/L and R Algorithm 18 point/Compute R(m) for 1 to 6/Compute R(m)_3 ==
  z : Inport
  zvalid : Inport  Port=2
  Add3 : Sum  Inputs=++|  OutDataTypeStr=Inherit: Inherit via back propagation
  Compare To Constant : simulink/Logic and Bit Operations/Compare To Constant  relop=>=  const=m  OutDataTypeStr=boolean
  Compare To Constant2 : simulink/Logic and Bit Operations/Compare To Constant  relop===  const=N - 1  OutDataTypeStr=boolean
  Complex Multiplier : Subsystem  VariantControl=Use 3 multipliers and 5 adders
      mask Display: disp(['Complex Multiplier' newline 'Latency = 8']);
  Data Type Duplicate : DataTypeDuplicate
  Data Type Conversion : DataTypeConversion  Commented=through  OutDataTypeStr=fixdt(1,28,17)  SaturateOnIntegerOverflow=off  RndMeth=Floor
  Delay : Delay  DelayLength=m
  Delay{1..2,7..9,11..12,14..15} (9 alike) : Delay  DelayLength=1
  Delay{3..6,10,13,16..26} (17 alike) : Delay
  Delay{27..30} (4 alike) : Delay  DelayLength=8
  Gain : Gain  Gain=MulDivFactor  ParamDataTypeStr=Inherit: Inherit from 'Gain'  OutDataTypeStr=Inherit: Same as input
  HDL Counter : hdlsllib/Sources/HDL Counter  CountType=Count limited  CountInit=0  CountStep=1  CountMax=N-1  CountFromType=Initial value  CountFrom=0  CountResetPort=off  CountLoadPort=off  CountEnbPort=on  CountDirPort=off  CountHitOutputPort=off  CountDataType=Unsigned  CountWordLen=nextpow2(N-1)  CountFracLen=0  CountSampTime=1
  Logical Operator : Logic  AllPortsSameDT=off  OutDataTypeStr=boolean
  Logical Operator1 : Logic  AllPortsSameDT=off  OutDataTypeStr=boolean
  Math Function : Math  Operator=conj
  Unit Delay Enabled Synchronous : hdlsllib/Discrete/Unit Delay Enabled Synchronous  InitialCondition=0.0  SampleTime=-1
  Unit Delay Enabled Resettable Synchronous : hdlsllib/Discrete/Unit Delay Enabled Resettable Synchronous  InitialCondition=0.0  SampleTime=-1
  Out1 : Outport
  wires:
  Data Type Conversion/1 -> Delay13/1
  Delay30/1 -> Delay20/1
  Delay29/1 -> Compare To Constant2/1
  Delay28/1 -> Compare To Constant/1
  Delay27/1 -> Delay17/1
  Delay13/1 -> Delay21/1
  Complex Multiplier/1(Out1) -> Data Type Conversion/1
  Delay26/1 -> Delay1/1
  Logical Operator/1 -> Delay25/1
  Delay24/1 -> Unit Delay Enabled Resettable Synchronous/2
  Delay23/1 -> Delay24/1
  Delay22/1 -> Add3/2, Data Type Duplicate/1
  Delay21/1 -> Gain/1
  Gain/1 -> Delay22/1
  Unit Delay Enabled Synchronous/1 -> Out1/1
  Delay20/1 -> Logical Operator/2
  Delay19/1 -> Logical Operator/1
  Delay18/1 -> Logical Operator1/2
  Delay17/1 -> Logical Operator1/1
  Delay16/1 -> Delay30/1
  Delay15/1 -> Delay16/1
  Delay12/1 -> Delay6/1
  Delay11/1 -> Delay5/1
  Delay10/1 -> Delay27/1
  Delay9/1 -> Delay10/1
  Delay8/1 -> Delay4/1
  Delay7/1 -> Delay3/1
  Delay6/1 -> Delay29/1
  Delay5/1 -> Delay28/1
  Delay4/1 -> Complex Multiplier/2(In2)
  Delay3/1 -> Complex Multiplier/1(In1)
  Delay2/1 -> Delay/1, Delay7/1
  Delay14/1 -> HDL Counter/1, Delay15/1, Delay9/1
  Math Function/1 -> Delay8/1
  z/1 -> Delay2/1
  Delay/1 -> Math Function/1
  Delay1/1 -> Unit Delay Enabled Resettable Synchronous/3, Unit Delay Enabled Synchronous/2
  Unit Delay Enabled Resettable Synchronous/1 -> Add3/1, Unit Delay Enabled Synchronous/1
  zvalid/1 -> Delay14/1
  Delay25/1 -> Delay26/1
  Compare To Constant2/1 -> Delay19/1
  Compare To Constant/1 -> Delay18/1
  HDL Counter/1 -> Delay12/1, Delay11/1
  Add3/1 -> Unit Delay Enabled Resettable Synchronous/1, Data Type Duplicate/2
  Logical Operator1/1 -> Delay23/1

== system soc_dvbs2_fpga/DVBS2/DVBS2 TxRx/DVB-S2 HDL Receiver/Synchronizer and PL Header Decoder/Time Frequency and Coarse Phase Synchronizer/Fine Frequency Synchronizer/Modified L and R Algorithm/L and R Algorithm 18 point/Compute R(m) for 1 to 6/Compute R(m)_4 ==
  z : Inport
  zvalid : Inport  Port=2
  Add3 : Sum  Inputs=++|  OutDataTypeStr=Inherit: Inherit via back propagation
  Compare To Constant : simulink/Logic and Bit Operations/Compare To Constant  relop=>=  const=m  OutDataTypeStr=boolean
  Compare To Constant2 : simulink/Logic and Bit Operations/Compare To Constant  relop===  const=N - 1  OutDataTypeStr=boolean
  Complex Multiplier : Subsystem  VariantControl=Use 3 multipliers and 5 adders
      mask Display: disp(['Complex Multiplier' newline 'Latency = 8']);
  Data Type Duplicate : DataTypeDuplicate
  Data Type Conversion : DataTypeConversion  Commented=through  OutDataTypeStr=fixdt(1,28,17)  SaturateOnIntegerOverflow=off  RndMeth=Floor
  Delay : Delay  DelayLength=m
  Delay{1..2,7..9,11..12,14..15} (9 alike) : Delay  DelayLength=1
  Delay{3..6,10,13,16..26} (17 alike) : Delay
  Delay{27..30} (4 alike) : Delay  DelayLength=8
  Gain : Gain  Gain=MulDivFactor  ParamDataTypeStr=Inherit: Inherit from 'Gain'  OutDataTypeStr=Inherit: Same as input
  HDL Counter : hdlsllib/Sources/HDL Counter  CountType=Count limited  CountInit=0  CountStep=1  CountMax=N-1  CountFromType=Initial value  CountFrom=0  CountResetPort=off  CountLoadPort=off  CountEnbPort=on  CountDirPort=off  CountHitOutputPort=off  CountDataType=Unsigned  CountWordLen=nextpow2(N-1)  CountFracLen=0  CountSampTime=1
  Logical Operator : Logic  AllPortsSameDT=off  OutDataTypeStr=boolean
  Logical Operator1 : Logic  AllPortsSameDT=off  OutDataTypeStr=boolean
  Math Function : Math  Operator=conj
  Unit Delay Enabled Synchronous : hdlsllib/Discrete/Unit Delay Enabled Synchronous  InitialCondition=0.0  SampleTime=-1
  Unit Delay Enabled Resettable Synchronous : hdlsllib/Discrete/Unit Delay Enabled Resettable Synchronous  InitialCondition=0.0  SampleTime=-1
  Out1 : Outport
  wires:
  Data Type Conversion/1 -> Delay13/1
  Logical Operator1/1 -> Delay23/1
  Add3/1 -> Data Type Duplicate/2, Unit Delay Enabled Resettable Synchronous/1
  HDL Counter/1 -> Delay11/1, Delay12/1
  Compare To Constant/1 -> Delay18/1
  Compare To Constant2/1 -> Delay19/1
  Delay25/1 -> Delay26/1
  zvalid/1 -> Delay14/1
  Unit Delay Enabled Resettable Synchronous/1 -> Unit Delay Enabled Synchronous/1, Add3/1
  Delay1/1 -> Unit Delay Enabled Synchronous/2, Unit Delay Enabled Resettable Synchronous/3
  Delay/1 -> Math Function/1
  z/1 -> Delay2/1
  Math Function/1 -> Delay8/1
  Delay14/1 -> Delay9/1, Delay15/1, HDL Counter/1
  Delay2/1 -> Delay7/1, Delay/1
  Delay3/1 -> Complex Multiplier/1(In1)
  Delay4/1 -> Complex Multiplier/2(In2)
  Delay5/1 -> Delay28/1
  Delay6/1 -> Delay29/1
  Delay7/1 -> Delay3/1
  Delay8/1 -> Delay4/1
  Delay9/1 -> Delay10/1
  Delay10/1 -> Delay27/1
  Delay11/1 -> Delay5/1
  Delay12/1 -> Delay6/1
  Delay15/1 -> Delay16/1
  Delay16/1 -> Delay30/1
  Delay17/1 -> Logical Operator1/1
  Delay18/1 -> Logical Operator1/2
  Delay19/1 -> Logical Operator/1
  Delay20/1 -> Logical Operator/2
  Unit Delay Enabled Synchronous/1 -> Out1/1
  Gain/1 -> Delay22/1
  Delay21/1 -> Gain/1
  Delay22/1 -> Data Type Duplicate/1, Add3/2
  Delay23/1 -> Delay24/1
  Delay24/1 -> Unit Delay Enabled Resettable Synchronous/2
  Logical Operator/1 -> Delay25/1
  Delay26/1 -> Delay1/1
  Complex Multiplier/1(Out1) -> Data Type Conversion/1
  Delay13/1 -> Delay21/1
  Delay27/1 -> Delay17/1
  Delay28/1 -> Compare To Constant/1
  Delay29/1 -> Compare To Constant2/1
  Delay30/1 -> Delay20/1

== system soc_dvbs2_fpga/DVBS2/DVBS2 TxRx/DVB-S2 HDL Receiver/Synchronizer and PL Header Decoder/Time Frequency and Coarse Phase Synchronizer/Fine Frequency Synchronizer/Modified L and R Algorithm/L and R Algorithm 18 point/Compute R(m) for 1 to 6/Compute R(m)_5 ==
  z : Inport
  zvalid : Inport  Port=2
  Add3 : Sum  Inputs=++|  OutDataTypeStr=Inherit: Inherit via back propagation
  Compare To Constant : simulink/Logic and Bit Operations/Compare To Constant  relop=>=  const=m  OutDataTypeStr=boolean
  Compare To Constant2 : simulink/Logic and Bit Operations/Compare To Constant  relop===  const=N - 1  OutDataTypeStr=boolean
  Complex Multiplier : Subsystem  VariantControl=Use 3 multipliers and 5 adders
      mask Display: disp(['Complex Multiplier' newline 'Latency = 8']);
  Data Type Duplicate : DataTypeDuplicate
  Data Type Conversion : DataTypeConversion  Commented=through  OutDataTypeStr=fixdt(1,28,17)  SaturateOnIntegerOverflow=off  RndMeth=Floor
  Delay : Delay  DelayLength=m
  Delay{1..2,7..9,11..12,14..15} (9 alike) : Delay  DelayLength=1
  Delay{3..6,10,13,16..26} (17 alike) : Delay
  Delay{27..30} (4 alike) : Delay  DelayLength=8
  Gain : Gain  Gain=MulDivFactor  ParamDataTypeStr=Inherit: Inherit from 'Gain'  OutDataTypeStr=Inherit: Same as input
  HDL Counter : hdlsllib/Sources/HDL Counter  CountType=Count limited  CountInit=0  CountStep=1  CountMax=N-1  CountFromType=Initial value  CountFrom=0  CountResetPort=off  CountLoadPort=off  CountEnbPort=on  CountDirPort=off  CountHitOutputPort=off  CountDataType=Unsigned  CountWordLen=nextpow2(N-1)  CountFracLen=0  CountSampTime=1
  Logical Operator : Logic  AllPortsSameDT=off  OutDataTypeStr=boolean
  Logical Operator1 : Logic  AllPortsSameDT=off  OutDataTypeStr=boolean
  Math Function : Math  Operator=conj
  Unit Delay Enabled Synchronous : hdlsllib/Discrete/Unit Delay Enabled Synchronous  InitialCondition=0.0  SampleTime=-1
  Unit Delay Enabled Resettable Synchronous : hdlsllib/Discrete/Unit Delay Enabled Resettable Synchronous  InitialCondition=0.0  SampleTime=-1
  Out1 : Outport
  wires:
  Data Type Conversion/1 -> Delay13/1
  Delay30/1 -> Delay20/1
  Delay29/1 -> Compare To Constant2/1
  Delay28/1 -> Compare To Constant/1
  Delay27/1 -> Delay17/1
  Delay13/1 -> Delay21/1
  Complex Multiplier/1(Out1) -> Data Type Conversion/1
  Delay26/1 -> Delay1/1
  Logical Operator/1 -> Delay25/1
  Delay24/1 -> Unit Delay Enabled Resettable Synchronous/2
  Delay23/1 -> Delay24/1
  Delay22/1 -> Add3/2, Data Type Duplicate/1
  Delay21/1 -> Gain/1
  Gain/1 -> Delay22/1
  Unit Delay Enabled Synchronous/1 -> Out1/1
  Delay20/1 -> Logical Operator/2
  Delay19/1 -> Logical Operator/1
  Delay18/1 -> Logical Operator1/2
  Delay17/1 -> Logical Operator1/1
  Delay16/1 -> Delay30/1
  Delay15/1 -> Delay16/1
  Delay12/1 -> Delay6/1
  Delay11/1 -> Delay5/1
  Delay10/1 -> Delay27/1
  Delay9/1 -> Delay10/1
  Delay8/1 -> Delay4/1
  Delay7/1 -> Delay3/1
  Delay6/1 -> Delay29/1
  Delay5/1 -> Delay28/1
  Delay4/1 -> Complex Multiplier/2(In2)
  Delay3/1 -> Complex Multiplier/1(In1)
  Delay2/1 -> Delay/1, Delay7/1
  Delay14/1 -> HDL Counter/1, Delay15/1, Delay9/1
  Math Function/1 -> Delay8/1
  z/1 -> Delay2/1
  Delay/1 -> Math Function/1
  Delay1/1 -> Unit Delay Enabled Resettable Synchronous/3, Unit Delay Enabled Synchronous/2
  Unit Delay Enabled Resettable Synchronous/1 -> Add3/1, Unit Delay Enabled Synchronous/1
  zvalid/1 -> Delay14/1
  Delay25/1 -> Delay26/1
  Compare To Constant2/1 -> Delay19/1
  Compare To Constant/1 -> Delay18/1
  HDL Counter/1 -> Delay12/1, Delay11/1
  Add3/1 -> Unit Delay Enabled Resettable Synchronous/1, Data Type Duplicate/2
  Logical Operator1/1 -> Delay23/1

== system soc_dvbs2_fpga/DVBS2/DVBS2 TxRx/DVB-S2 HDL Receiver/Synchronizer and PL Header Decoder/Time Frequency and Coarse Phase Synchronizer/Fine Frequency Synchronizer/Modified L and R Algorithm/L and R Algorithm 18 point/Compute R(m) for 1 to 6/Compute R(m)_6 ==
  z : Inport
  zvalid : Inport  Port=2
  Add3 : Sum  Inputs=++|  OutDataTypeStr=Inherit: Inherit via back propagation
  Compare To Constant : simulink/Logic and Bit Operations/Compare To Constant  relop=>=  const=m  OutDataTypeStr=boolean
  Compare To Constant2 : simulink/Logic and Bit Operations/Compare To Constant  relop===  const=N - 1  OutDataTypeStr=boolean
  Complex Multiplier : Subsystem  VariantControl=Use 3 multipliers and 5 adders
      mask Display: disp(['Complex Multiplier' newline 'Latency = 8']);
  Data Type Duplicate : DataTypeDuplicate
  Data Type Conversion : DataTypeConversion  Commented=through  OutDataTypeStr=fixdt(1,28,17)  SaturateOnIntegerOverflow=off  RndMeth=Floor
  Delay : Delay  DelayLength=m
  Delay{1..2,7..9,11..12,14..15} (9 alike) : Delay  DelayLength=1
  Delay{3..6,10,13,16..26} (17 alike) : Delay
  Delay{27..30} (4 alike) : Delay  DelayLength=8
  Gain : Gain  Gain=MulDivFactor  ParamDataTypeStr=Inherit: Inherit from 'Gain'  OutDataTypeStr=Inherit: Same as input
  HDL Counter : hdlsllib/Sources/HDL Counter  CountType=Count limited  CountInit=0  CountStep=1  CountMax=N-1  CountFromType=Initial value  CountFrom=0  CountResetPort=off  CountLoadPort=off  CountEnbPort=on  CountDirPort=off  CountHitOutputPort=off  CountDataType=Unsigned  CountWordLen=nextpow2(N-1)  CountFracLen=0  CountSampTime=1
  Logical Operator : Logic  AllPortsSameDT=off  OutDataTypeStr=boolean
  Logical Operator1 : Logic  AllPortsSameDT=off  OutDataTypeStr=boolean
  Math Function : Math  Operator=conj
  Unit Delay Enabled Synchronous : hdlsllib/Discrete/Unit Delay Enabled Synchronous  InitialCondition=0.0  SampleTime=-1
  Unit Delay Enabled Resettable Synchronous : hdlsllib/Discrete/Unit Delay Enabled Resettable Synchronous  InitialCondition=0.0  SampleTime=-1
  Out1 : Outport
  wires:
  Data Type Conversion/1 -> Delay13/1
  Logical Operator1/1 -> Delay23/1
  Add3/1 -> Data Type Duplicate/2, Unit Delay Enabled Resettable Synchronous/1
  HDL Counter/1 -> Delay11/1, Delay12/1
  Compare To Constant/1 -> Delay18/1
  Compare To Constant2/1 -> Delay19/1
  Delay25/1 -> Delay26/1
  zvalid/1 -> Delay14/1
  Unit Delay Enabled Resettable Synchronous/1 -> Unit Delay Enabled Synchronous/1, Add3/1
  Delay1/1 -> Unit Delay Enabled Synchronous/2, Unit Delay Enabled Resettable Synchronous/3
  Delay/1 -> Math Function/1
  z/1 -> Delay2/1
  Math Function/1 -> Delay8/1
  Delay14/1 -> Delay9/1, Delay15/1, HDL Counter/1
  Delay2/1 -> Delay7/1, Delay/1
  Delay3/1 -> Complex Multiplier/1(In1)
  Delay4/1 -> Complex Multiplier/2(In2)
  Delay5/1 -> Delay28/1
  Delay6/1 -> Delay29/1
  Delay7/1 -> Delay3/1
  Delay8/1 -> Delay4/1
  Delay9/1 -> Delay10/1
  Delay10/1 -> Delay27/1
  Delay11/1 -> Delay5/1
  Delay12/1 -> Delay6/1
  Delay15/1 -> Delay16/1
  Delay16/1 -> Delay30/1
  Delay17/1 -> Logical Operator1/1
  Delay18/1 -> Logical Operator1/2
  Delay19/1 -> Logical Operator/1
  Delay20/1 -> Logical Operator/2
  Unit Delay Enabled Synchronous/1 -> Out1/1
  Gain/1 -> Delay22/1
  Delay21/1 -> Gain/1
  Delay22/1 -> Data Type Duplicate/1, Add3/2
  Delay23/1 -> Delay24/1
  Delay24/1 -> Unit Delay Enabled Resettable Synchronous/2
  Logical Operator/1 -> Delay25/1
  Delay26/1 -> Delay1/1
  Complex Multiplier/1(Out1) -> Data Type Conversion/1
  Delay13/1 -> Delay21/1
  Delay27/1 -> Delay17/1
  Delay28/1 -> Compare To Constant/1
  Delay29/1 -> Compare To Constant2/1
  Delay30/1 -> Delay20/1
